simulink model "PMSM_FOC"  (R2013b)
settings: Solver=ode45  StartTime=0.0  StopTime=0.2  RelTol=1e-3
PostLoadFcn:
  | PMSM_Params
undefined symbols (not defined in the file or in its folder): Params, Plot_PMSM
libraries: powerlib x7, simulink x1
settings Model: Creator=Pascal  LastModifiedBy=reynaudp
settings OptimizationCC: OptimizeModelRefInitCode=on  LifeSpan=1
settings DebuggingCC: StateNameClashWarn=warning
settings HardwareCC: ProdLargestAtomicInteger=Integer  ProdLargestAtomicFloat=Float  ProdIntDivRoundTo=Zero  ProdEndianess=LittleEndian  ProdHWDeviceType=STMicroelectronics->STM32F4xx 32-bit Cortex-M4
settings RTWCC: SystemTargetFile=stm32F4xx.tlc  TemplateMakefile=stm32F4xx.tmf  Description=stm32F4xx (Embedded Target)  GenerateReport=on  ProcessScript=stm32F4xx_make_rtw_hook  LaunchReport=on  CodeExecutionProfiling=on  CodeProfilingSaveOptions=AllData  GenerateCodeReplacementReport=on
settings CodeAppCC: IgnoreCustomStorageClasses=off
settings STFCustomTargetCC: CodeReplacementLibrary=ARM CMSIS 3.01  ParMdlRefBuildCompliant=on  IncludeMdlTerminateFcn=off  CombineOutputUpdateFcns=on  ERTCustomFileBanners=on  SupportContinuousTime=off  SupportNonInlinedSFcns=off  MATLABClassNameForMDSCustomization=Simulink.SoftwareTarget.ERTCustomization  GRTInterface=off  SystemTargetFile=stm32F4xx.tlc
settings ERTTargetCC: CodeReplacementLibrary=ARM CMSIS 3.01  CompOptLevelCompliant=off  ConcurrentExecutionCompliant=off  IncludeMdlTerminateFcn=off  ERTFirstTimeCompliant=off  ModelStepFunctionPrototypeControlCompliant=off  CPPClassGenCompliant=off  InlinedParameterPlacement=NonHierarchical  ERTSrcFileBannerTemplate=sourceFileTemplate.cgt  ERTHdrFileBannerTemplate=sourceFileTemplate.cgt  ERTDataSrcFileTemplate=sourceFileTemplate.cgt  ERTDataHdrFileTemplate=sourceFileTemplate.cgt  ERTCustomFileTemplate=customRoutineProcess.tlc

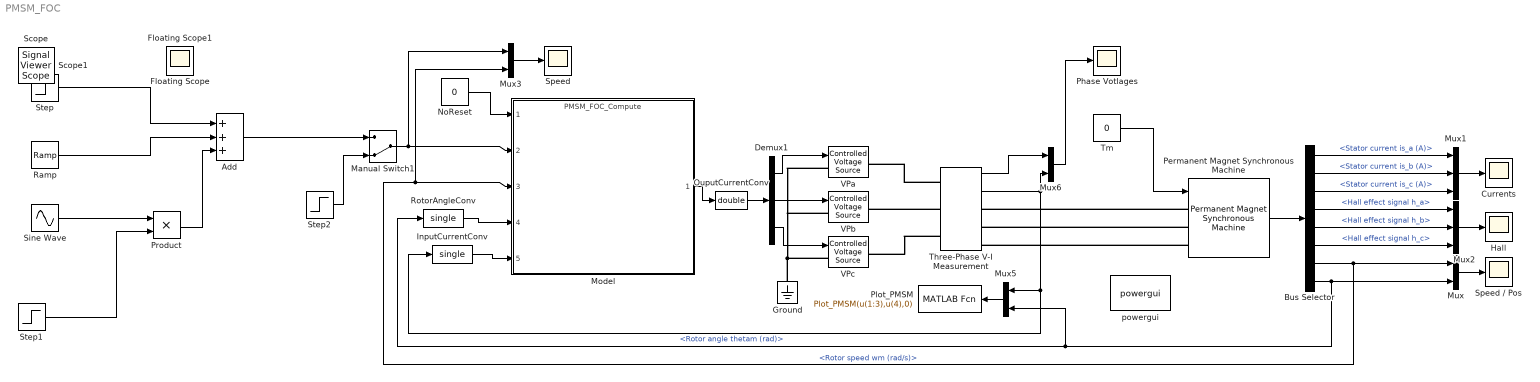
== system PMSM_FOC ==
  Add : Sum  Inputs=+++
  Bus Selector : BusSelector  OutputSignals=Stator current is_a (A),Stator current is_b (A),Stator current is_c (A),Hall effect signal h_a,Hall effect signal h_b,Hall effect signal h_c,Rotor speed wm (rad/s),Rotor angle thetam (rad)
  Currents : Scope
      settings: YMin=-0.4  YMax=0.4  SaveName=ScopeData3
  Demux1 : Demux  Outputs=3
  Ground : powerlib/Elements/Ground  LConnTagsString=a
  Hall : Scope
      settings: ShowLegends=on  TimeRange=1  YMin=0  YMax=1  SaveName=ScopeData2
  InputCurrentConv : DataTypeConversion  OutDataTypeStr=single
  Manual Switch1 : ManualSwitch  CurrentSetting=0
  Model : ModelReference  ModelNameDialog=PMSM_FOC_Compute.slx  SimulationMode=Normal  ModelReferenceVersion=1.77  CopyOfModelName=PMSM_FOC_Compute.slx  DefaultDataLogging=on
  Mux{,3,5..6} (4 alike) : Mux  Inputs=2
  Mux1 : Mux  Inputs=3
  Mux2 : Mux  Inputs=3
  NoReset : Constant  Value=0  OutDataTypeStr=boolean
  OuputCurrentConv : DataTypeConversion  OutDataTypeStr=double
  Permanent Magnet Synchronous Machine : powerlib/Machines/Permanent Magnet Synchronous Machine  NbPhases=3  FluxDistribution=Sinusoidal  RotorType=Round  MechanicalLoad=Torque Tm  PresetModel=No  ShowDetailedParameters=on  Resistance=.6  Inductance=1.4e-3  dqInductances=[6e-4,6e-4]  La=1.4e-3  MachineConstant=Voltage Constant (V_peak L-L / krpm)  Flux=0.034182  VoltageCst=6.2  TorqueCst=0.051274  Flat=120  Mechanical=[1.1e-5,1e-4,1,0.02]  PolePairs=1  InitialConditions=[0,0 0,0]  InitialConditions5ph=[0 0 0 0 0 0]  TsPowergui=0  TsBlock=-1  RefAngle=Aligned with phase A axis (original Park)
  Phase Votlages : Scope
      settings: YMin=-5.5  YMax=6
  Plot_PMSM : MATLABFcn  MATLABFcn=Plot_PMSM(u(1:3),u(4),0)  OutputDimensions=0  SampleTime=1/100
  Product : Product  RndMeth=Zero
  Ramp : simulink/Sources/Ramp  slope=50  start=2  X0=0
  RotorAngleConv : DataTypeConversion  OutDataTypeStr=single
  Sine Wave : Sin  Amplitude=20  Frequency=2*pi  SampleTime=0
  Speed : Scope
      settings: YMin=-10  YMax=150  SaveName=ScopeData6  MaxDataPoints=20000
  Speed / Pos : Scope
      settings: ShowLegends=on  TimeRange=8  YMin=-250  YMax=450
  Step : Step  Time=0.5  Before=-50  After=-80  SampleTime=0
  Step1 : Step  Time=4  SampleTime=0
  Step2 : Step  Time=.01  After=130  SampleTime=0
  Three-Phase V-I Measurement : powerlib/Measurements/Three-Phase V-I Measurement  VoltageMeasurement=phase-to-ground  SetLabelV=off  LabelV=Vabc  Vpu=off  VpuLL=off  CurrentMeasurement=yes  SetLabelI=off  LabelI=Iabc  Ipu=off  Pbase=100e6  Vbase=500e3  OutputType=Complex  PhasorSimulation=off  PSBequivalent=0
  Tm : Constant  Value=0
  VPa : powerlib/Electrical Sources/Controlled Voltage Source  Initialize=on  Source_Type=AC  Amplitude=0  Phase=0  Frequency=0  Measurements=None
  VPb : powerlib/Electrical Sources/Controlled Voltage Source  Initialize=on  Source_Type=AC  Amplitude=0  Phase=0  Frequency=0  Measurements=None
  VPc : powerlib/Electrical Sources/Controlled Voltage Source  Initialize=on  Source_Type=AC  Amplitude=0  Phase=0  Frequency=0  Measurements=None
  powergui : powerlib/powergui  Priority=1  SimulationMode=Discrete  SolverType=Tustin  SampleTime=Params.T  frequency=60  SPID=off  DisableSnubberDevices=off  DisableRonSwitches=off  DisableVfSwitches=off  SwTol=0  Interpol=off  DisplayEquations=off  frequencyindice=0  Pbase=100e6  ErrMax=1e-4  Iterations=50  UnitsV=kV  UnitsW=MW  FunctionMessages=off  echomessages=off  HookPort=off  EnableUseOfTLC=off  x0status=blocks  RestoreLinks=warning  ResistiveCurrentMeasurement=off  Frange=[0:2:500]  Ylog=off  Xlog=on  ShowGrid=off  save=off  variable=ZData  ZoomFFT=off  StartTime=0.0  cycles=1  DisplayStyle=1  fundamental=60  FreqAxis=off  MaxFrequency=1000  frequencyindicesteady=1  RmsSteady=1  display=off  Ts=0  methode=off
  Floating Scope : Scope
      settings: Floating=on  YMin=-100  YMax=325  SaveName=ScopeData4
  Floating Scope1 : Scope
      settings: Floating=on  YMin=-100  YMax=60  SaveName=ScopeData5
  Scope : SignalViewerScope  IOType=viewer  RefreshTime=0.035000
      settings: YMin=265  YMax=320
  Scope1 : SignalViewerScope  IOType=viewer  RefreshTime=0.035000
      settings: YMin=-100  YMax=175
  wires:
  Step/1 -> Add/1
  Ramp/1 -> Add/2
  Sine Wave/1 -> Product/1
  Step1/1 -> Product/2
  Product/1 -> Add/3
  Add/1 -> Manual Switch1/1
  Step2/1 -> Manual Switch1/2
  Demux1/1 -> VPa/1
  Demux1/2 -> VPb/1
  Demux1/3 -> VPc/1
  Model/1 -> OuputCurrentConv/1
  Tm/1 -> Permanent Magnet Synchronous Machine/1
  Three-Phase V-I Measurement/1 -> Mux6/1
  Mux6/1 -> Phase Votlages/1
  Bus Selector/1 -> Mux1/1  "<Stator current is_a (A)>"
  Bus Selector/2 -> Mux1/2  "<Stator current is_b (A)>"
  Bus Selector/3 -> Mux1/3  "<Stator current is_c (A)>"
  Mux1/1 -> Currents/1
  Bus Selector/7 -> Mux3/2, Model/3, Mux/1  "<Rotor speed wm (rad/s)>"
  Bus Selector/4 -> Mux2/1  "<Hall effect signal h_a>"
  Bus Selector/5 -> Mux2/2  "<Hall effect signal h_b>"
  Bus Selector/6 -> Mux2/3  "<Hall effect signal h_c>"
  Mux2/1 -> Hall/1
  Mux/1 -> Speed / Pos/1
  Permanent Magnet Synchronous Machine/1 -> Bus Selector/1
  Mux3/1 -> Speed/1
  OuputCurrentConv/1 -> Demux1/1
  InputCurrentConv/1 -> Model/5
  RotorAngleConv/1 -> Model/4
  Manual Switch1/1 -> Model/2, Mux3/1
  NoReset/1 -> Model/1
  Bus Selector/8 -> Mux5/2, RotorAngleConv/1, Mux/2  "<Rotor angle thetam (rad)>"
  Three-Phase V-I Measurement/2 -> Mux6/2, InputCurrentConv/1, Mux5/1
  Mux5/1 -> Plot_PMSM/1
  connections:
  VPc/LConn1 -- VPa/LConn1 -- VPb/LConn1 -- Ground/LConn1
  Permanent Magnet Synchronous Machine/LConn1 -- Three-Phase V-I Measurement/RConn1
  Permanent Magnet Synchronous Machine/LConn2 -- Three-Phase V-I Measurement/RConn2
  Permanent Magnet Synchronous Machine/LConn3 -- Three-Phase V-I Measurement/RConn3
  Three-Phase V-I Measurement/LConn1 -- VPa/RConn1
  Three-Phase V-I Measurement/LConn2 -- VPb/RConn1
  Three-Phase V-I Measurement/LConn3 -- VPc/RConn1
